simulink model "musyndm2"  (Simulink 3.00)
settings: Solver=ode15s  SolverMode=SingleTasking  StartTime=0.0  StopTime=200  MaxStep=0.1  RelTol=1e-3  AbsTol=1e-6
PreLoadFcn:
  | mudata2
values from neighbouring files (symbols this model uses):
  bp = pimp(bnum)    [fitchose.m]
  cp = cumsum([1;sizecdA(:,1)+sizecdB(:,1)])    [mamilc.m]
  dp = cumsum([1;sizecdA(:,2)+sizecdB(:,2)])    [mamilc.m]
undefined symbols (not defined in the file or in its folder): ap, den_i, num_i
settings Model: ExternalInput=[]  SaveTime=off  SaveOutput=off  InitialState=[]  RTWTemplateMakefile=grt_vc.tmf  ExtModeMexFile=ext_comm.c  Creator=greg  LastModifiedBy=David High

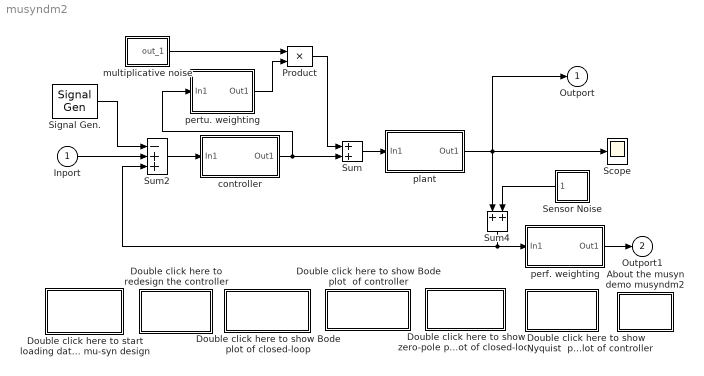
== system musyndm2 ==
  Inport : Inport  Port=1  PortWidth=-1  SampleTime=-1  DataType=auto
      settings: SignalType=auto
  About the musyn demo musyndm2 : Subsystem
      settings: OpenFcn=clc; more(24); help mudata2; more off;
      mask Display: disp('?')
  Double click here to redesign the controller : Subsystem
      settings: OpenFcn=if ~exist('a'),fprintf('\nMust load data first\n'), else, fprintf('\nPress Ctrl_C to abort MuSyn Calculation\n\n'); mudes2; end
      mask Display: disp('Re-design')
  Double click here to show Bode plot of closed-loop : Subsystem
      settings: OpenFcn=if ~exist('mu'),fprintf('\nMust be licensed for Mu Toolbox\n'),elseif ~exist('g1'),fprintf('\nMust Load Data & Design First\n'),else,eval('vplot(''bode'',frsp(g1,logspace(0,4,32)))');end
      mask Display: disp('Closed-Loop\nBode Plot')
  Double click here to show Bode plot  of controller : Subsystem
      settings: OpenFcn=if ~exist('mu'),fprintf('\nMust be licensed for Mu Toolbox\n'),elseif ~exist('k1'),fprintf('\nMust Load Data & Design First\n'),else,eval('vplot(''bode'',frsp(k1,logspace(0,4,32)))');end
      mask Display: disp('Controller\nBode Plot')
  Double click here to show Nyquist  plot of controller : Subsystem
      settings: OpenFcn=if ~exist('mu'),fprintf('\nMust be licensed for Mu Toolbox\n'),elseif ~exist('k1'),fprintf('\nMust Load Data & Design First\n'),else,omtt=logspace(-6,6,100);eval('foo=frsp(k1,omtt);foobar=frsp(k1,-omtt);');vplot('nyq',foo,foobar);end
      mask Display: disp('Controller\nNyquist')
  Double click here to show zero-pole plot of closed-loop : Subsystem
      settings: OpenFcn=if ~exist('mu'),fprintf('\nMust be licensed for Mu Toolbox\n'),elseif ~exist('g1'), fprintf('Must Load Data & Design First'), else,clf,plot(1:10), eval('[x,y,z,w]=unpck(g1);clf;pzmap(x,y,z,w);clear x y z w');end
      mask Display: disp('Controller\nZero-Pole Plot')
  Double click here to start loading data and mu-syn design : Subsystem
      settings: OpenFcn=if ~exist('mu'),fprintf('\nMust be licensed for MuSyn Toolbox\n'), else, fprintf('\nLoading Data\nWarning: New data will overlap the original working data\n>>\n'); mudata2; end
      mask Display: disp('Re-Load\nData')
  Product : Product  Inputs=2  SaturateOnIntegerOverflow=on
  Scope : Scope
      settings: TickLabels=on  TimeRange=10.000000  YMin=-5  YMax=5  SaveToWorkspace=off  SaveName=ScopeData  DataFormat=Matrix
  Sensor Noise : Subsystem  Orientation=left  mask{@1=0.01, @2=0.11, @3=23341}
      mask prompts: @1 "Noise Variance:"; @2 "Sample Time:"; @3 "Seed"
      mask help:
      | White noise for continuous (s-domain) systems.
      | Band-limited using zero-order-hold.
      mask init:
      | Cov = @1; Ts = @2; seed = @3; r = rand(1,12)-0.5; r2 = [r(1),r;r,r(12)]; t =[1:13;1:13];
      mask Help: Implemented using white noise into Zero Order Hold block. For faster simulation set sample time to highest value possible but in accordance with the fastest dynamics of system.
      mask Display: plot(t(:),r2(:))
  Signal Gen. : SignalGenerator  WaveForm=square  Amplitude=2.000000  Frequency=1.000000  Units=rad/sec
  Sum : Sum  Inputs=++  SaturateOnIntegerOverflow=on
  Sum2 : Sum  Inputs=-++  SaturateOnIntegerOverflow=on
  Sum4 : Sum  Orientation=down  Inputs=++  SaturateOnIntegerOverflow=on
  controller : Subsystem  mask{@1=ak, @2=bk, @3=ck, @4=dk}
      mask prompts: @1 "ak:"; @2 "bk:"; @3 "ck:"; @4 "dk:"
      mask help: H_infty Controller:
      mask init:
      | ak=@1;bk=@2;ck=@3;dk=@4;
      mask Help: . Mask and unmask this block to see how it works.Usinf Mu Analysis and Synthesis Toolbox to design a H_infinity Controller. Change the parameters, see the designed system.
      mask Display: disp('H_infinity\nController')
  multiplicative noise : Subsystem  mask{@1=0.1, @2=1, @3=68932234}
      mask prompts: @1 "Noise Variance:"; @2 "Sample Time:"; @3 "Seed"
      mask help:
      | White noise for continuous (s-domain) systems.
      | Band-limited using zero-order-hold.
      mask init:
      | Cov = @1; Ts = @2; seed = @3; r = rand(1,12)-0.5; r2 = [r(1),r;r,r(12)]; t =[1:13;1:13];
      mask Help: Implemented using white noise into Zero Order Hold block. For faster simulation set sample time to highest value possible but in accordance with the fastest dynamics of system.
      mask Display: plot(t(:),r2(:))
  perf. weighting : Subsystem  mask{@1=num_o, @2=den_o}
      mask prompts: @1 "numerator:"; @2 "denominator:"
      mask help: Performance weighting function:
      mask init:
      | [ap,bp,cp,dp]=tf2ss(@1,@2);
      mask Help: This is the weighting function of the plant model.
      mask Display: disp('output\nweighting.')
  pertu. weighting : Subsystem
      mask Type: Transfer Fcn
      mask Display: disp('   input   \nweighting')
  plant : Subsystem  mask{@1=a, @2=b, @3=c, @4=d}
      mask prompts: @1 "a:"; @2 "b:"; @3 "c:"; @4 "d:"
      mask help: state space model:
      mask init:
      | a=@1; b=@2; c=@3; d=@4;
      mask Help: system plant
      mask Display: disp('plant\nmodel')
  Outport : Outport  Port=1
  Outport1 : Outport  Port=2
  wires:
  plant/1(Out1) -> Scope/1, Outport/1, Sum4/1
  Sum2/1 -> controller/1(In1)
  Inport/1 -> Sum2/2
  perf. weighting/1(Out1) -> Outport1/1
  pertu. weighting/1(Out1) -> Product/2
  Sum/1 -> plant/1(In1)
  multiplicative noise/1(out_1) -> Product/1
  Sensor Noise/1(out_1) -> Sum4/2
  Signal Gen./1 -> Sum2/1
  Sum4/1 -> Sum2/3, perf. weighting/1(In1)
  Product/1 -> Sum/1
  controller/1(Out1) -> Sum/2, pertu. weighting/1(In1)

== system musyndm2/About the musyn demo musyndm2 ==

== system musyndm2/Double click here to redesign the controller ==

== system musyndm2/Double click here to show Bode plot of closed-loop ==

== system musyndm2/Double click here to show Bode plot  of controller ==

== system musyndm2/Double click here to show Nyquist  plot of controller ==

== system musyndm2/Double click here to show zero-pole plot of closed-loop ==

== system musyndm2/Double click here to start loading data and mu-syn design ==

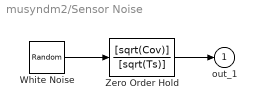
== system musyndm2/Sensor Noise ==
  White Noise : RandomNumber  Mean=0  Variance=1  Seed=seed  SampleTime=Ts
  Zero Order Hold : DiscreteTransferFcn  Numerator=[sqrt(Cov)]  Denominator=[sqrt(Ts)]  SampleTime=Ts
  out_1 : Outport  Port=1
  wires:
  White Noise/1 -> Zero Order Hold/1
  Zero Order Hold/1 -> out_1/1

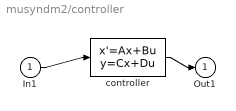
== system musyndm2/controller ==
  In1 : Inport  Port=1  PortWidth=-1  SampleTime=-1  DataType=auto
      settings: SignalType=auto
  controller : StateSpace  A=ak  B=bk  C=ck  D=dk  X0=0
  Out1 : Outport  Port=1
  wires:
  In1/1 -> controller/1
  controller/1 -> Out1/1

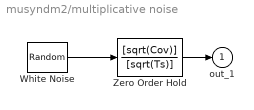
== system musyndm2/multiplicative noise ==
  White Noise : RandomNumber  Mean=0  Variance=1  Seed=seed  SampleTime=Ts
  Zero Order Hold : DiscreteTransferFcn  Numerator=[sqrt(Cov)]  Denominator=[sqrt(Ts)]  SampleTime=Ts
  out_1 : Outport  Port=1
  wires:
  Zero Order Hold/1 -> out_1/1
  White Noise/1 -> Zero Order Hold/1

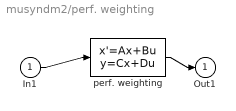
== system musyndm2/perf. weighting ==
  In1 : Inport  Port=1  PortWidth=-1  SampleTime=-1  DataType=auto
      settings: SignalType=auto
  perf. weighting : StateSpace  A=ap  B=bp  C=cp  D=dp  X0=0
  Out1 : Outport  Port=1
  wires:
  In1/1 -> perf. weighting/1
  perf. weighting/1 -> Out1/1

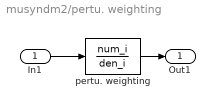
== system musyndm2/pertu. weighting ==
  In1 : Inport  Port=1  PortWidth=-1  SampleTime=-1  DataType=auto
      settings: SignalType=auto
  pertu. weighting : TransferFcn  Numerator=num_i  Denominator=den_i
  Out1 : Outport  Port=1
  wires:
  In1/1 -> pertu. weighting/1
  pertu. weighting/1 -> Out1/1

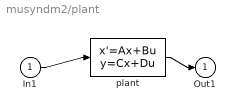
== system musyndm2/plant ==
  In1 : Inport  Port=1  PortWidth=-1  SampleTime=-1  DataType=auto
      settings: SignalType=auto
  plant : StateSpace  A=a  B=b  C=c  D=d  X0=0
  Out1 : Outport  Port=1
  wires:
  In1/1 -> plant/1
  plant/1 -> Out1/1
